simulink model "psi_model"  (R2016b)
settings: Solver=ode4  StartTime=0.0  StopTime=1  FixedStep=0.02  RelTol=1e-3
values from neighbouring files (symbols this model uses):
  rho3 = x(1)    [leastSquare.m]
  rho4 = x(2)    [leastSquare.m]
settings Model: Creator=Ernie  LastModifiedBy=Ernie

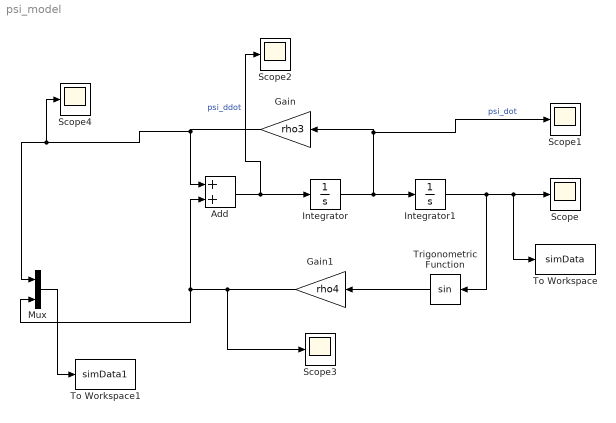
== system psi_model ==
  Add : Sum
  Gain : Gain  Gain=rho3
  Gain1 : Gain  Gain=rho4
  Integrator : Integrator  InitialCondition=0.0055
  Integrator1 : Integrator  InitialCondition=0.0012
  Mux : Mux  Inputs=2
  Scope{,1..4} (5 alike) : Scope
  To Workspace : ToWorkspace  VariableName=simData  SaveFormat=Timeseries  SampleTime=-1
  To Workspace1 : ToWorkspace  VariableName=simData1  SaveFormat=Timeseries  SampleTime=-1
  Trigonometric Function : Trigonometry
  wires:
  Integrator/1 -> Scope1/1, Gain/1, Integrator1/1  "psi_dot"
  Add/1 -> Scope2/1, Integrator/1  "psi_ddot"
  Gain/1 -> Mux/1, Scope4/1, Add/1
  Integrator1/1 -> To Workspace/1, Scope/1, Trigonometric Function/1
  Trigonometric Function/1 -> Gain1/1
  Gain1/1 -> Scope3/1, Mux/2, Add/2
  Mux/1 -> To Workspace1/1
